simulink model "ee_synrm_torque_control_v1"  (R2023a)
settings: Solver=FixedStepDiscrete  StartTime=0.0  StopTime=1.5  FixedStep=Ts  RelTol=1e-3  EnableMultiTasking=on
PreLoadFcn:
  | ee_synrm_torque_control_data;
StopFcn:
  | ee_addSimlogTimeStamp(bdroot)
undefined symbols (not defined in the file): Ld, Lq, p, Ts
libraries: nesl_utility x13, fl_lib x9, ee_lib x4, eeTransforms x2, eePmsmCurrentController x1, simulink x1, eePwmGeneratorTwoLevel x1, batteryecm_lib x1, SignalEditorBlockLib x1
CloseFcn:
  | clear simlog_ee_synrm_torque_control
  | clear logsout_ee_synrm_torque_control
Description:
  | Synchronous Reluctance Machine Torque Control
settings Model: Creator=The MathWorks, Inc.  LastModifiedBy=ravikrishna_g3
settings SolverCC: AlgebraicLoopSolver=TrustRegion  MaxZcPerStep=1
settings DataIOCC: MaxDataPoints=310000  ReturnWorkspaceOutputs=off  SignalLoggingName=logsout_ee_synrm_torque_control
settings OptimizationCC: ReuseModelBlockBuffer=off  LifeSpan=inf
settings DebuggingCC: UnderspecifiedInitializationDetection=Classic  MergeDetectMultiDrivingBlocksExec=none  UnconnectedInputMsg=warning  UnconnectedOutputMsg=warning  UnconnectedLineMsg=warning  SFUnexpectedBacktrackingDiag=warning  SFNoUnconditionalDefaultTransitionDiag=warning  SFExecutionAtInitializationDiag=none  ArithmeticOperatorsInVariantConditions=warning
settings ModelReferenceCC: EnableRefExpFcnMdlSchedulingChecks=on
settings SFSimCC: SimUseLocalCustomCode=off  CustomCodeUndefinedFunction=UseInterfaceOnly
settings RTWCC: RTWUseLocalCustomCode=off  DLArmComputeVersion=19.05
settings CodeAppCC: StateflowObjectComments=on
settings GRTTargetCC: TargetLangStandard=C89/C90 (ANSI)
settings ConfigComp: CovMetricSettings=dw  CovSaveCumulativeToWorkspaceVar=on  CovSaveSingleToWorkspaceVar=on  CovExternalEMLEnable=off
settings SimscapeCC: SimscapeLogType=all  SimscapeLogSimulationStatistics=on  SimscapeLogName=simlog_ee_synrm_torque_control  SimscapeLogDataHistory=310000

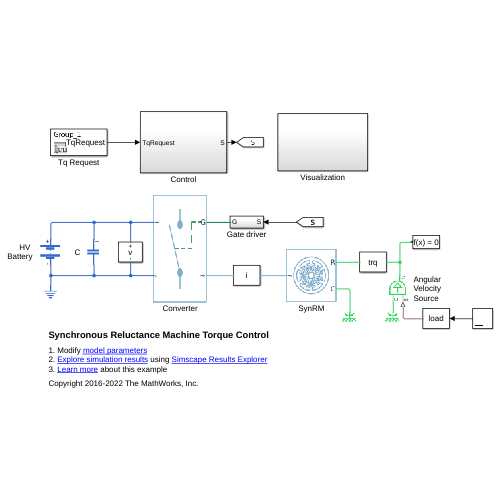
[thumbnail: Simulink's stored preview of the top-level diagram]
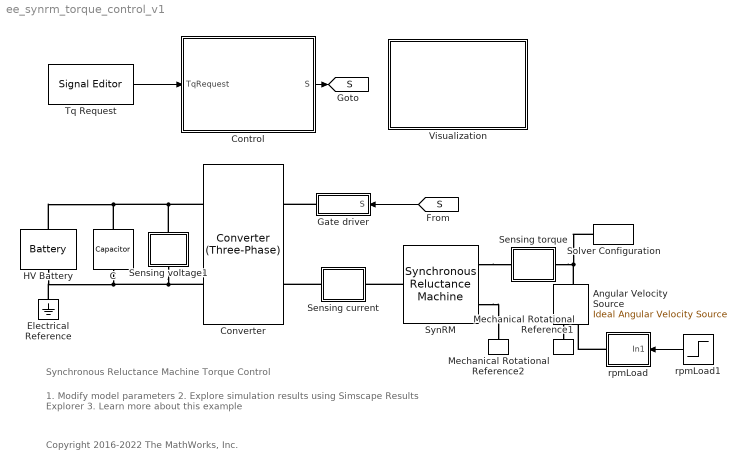
== system ee_synrm_torque_control_v1 ==
  note: Synchronous Reluctance Machine Torque Control
  note: 1. Modify model parameters
      | 2. Explore simulation results using Simscape Results Explorer
      | 3. Learn more about this example
  note: Copyright 2016-2022 The MathWorks, Inc.
  Angular Velocity Source : fl_lib/Mechanical/Mechanical Sources/Ideal Angular Velocity Source
  C : fl_lib/Electrical/Electrical Elements/Capacitor  c=Cdc F  r=1e-6 Ohm  g=0 1/Ohm  i_specify=off  i_priority=None  i=0 A  i_nominal_specify=off  i_nominal_unit=A  i_nominal_value=1  v_specify=off  v_priority=None  v=0 V  v_nominal_specify=off  v_nominal_unit=V  v_nominal_value=1  vc_specify=on  vc_priority=None  vc=Vnom V  vc_nominal_specify=off  vc_nominal_unit=V  vc_nominal_value=1
  Control : Subsystem
  Converter : ee_lib/Semiconductors & Converters/Converters/Converter (Three-Phase)  port_option=ee.enum.threePhasePort.composite  device_type=3  K=0  Vf=0.8 V  Ron=0.001 Ohm  Rds=0.001 Ohm  Goff=1e-5 1/Ohm  Vgt=1 V  Vgt_off=-1 V  Ih=1 A  Vth=0.5 V  diode_param=2  diode_Vf=0.8 V  diode_Ron=0.001 Ohm  diode_Goff=1e-5 1/Ohm  diode_C=50 nF  diode_iRM=-235 A  diode_iF=300 A  diode_idot=-50 A/us  diode_trr_param=1  diode_trr_factor=3  diode_trr=15 us  diode_Qrr=1.5e+3 s*uA  snubber_type=0  Cs=1e-7 F  Rs=0.1 Ohm
  Electrical Reference : fl_lib/Electrical/Electrical Elements/Electrical Reference
  Gate driver : Subsystem
  HV Battery : batteryecm_lib/Battery  Vnom=Vnom V  prm_dir=1  R1_dis=2 Ohm  R1_ch=2 Ohm  R1=0.001 Ohm  prm_AH=1  AH=10000 hr*A  V1=V1 V  AH1=3000 hr*A  prm_R2=1  R2=2000 Ohm  Tmeas=298.15 K  charge_measurement_port=simscape.enum.battery.enable.no  prm_dyn=1  Rp1=0.005 Ohm  tau1=30 s  Rp2=0.005 Ohm  tau2=30 s  Rp3=0.005 Ohm  tau3=30 s  Rp4=0.005 Ohm  tau4=30 s  Rp5=0.005 Ohm  tau5=30 s  prm_fade=1  N_fade=100  AH_fade=45 hr*A  R1_fade=2.02 Ohm  R1_ch_fade=2.02 Ohm  V1_fade=10.35 V  prm_age=1  prm_age_OCV=1  OCV_age=0.9  SOC_age=60  Tmeas_age=298.15 K  delta_time_age_vec=[0] d  temperature_age_vec=[273] K  OCV_scaling_age=2.2134e6  OCV_offset_age=1.632e6  temp_exp_age=0.515833569 V  t_exp_age=0.75  Vnom_T2=12 V  R1_T2=2.2 Ohm  R1_T2_dis=2.2 Ohm  R1_T2_ch=2.2 Ohm  V1_T2=11.4 V  R2_T2=2200 Ohm  Rp1_T2=0.005 Ohm  tau1_T2=30 s  Rp2_T2=0.005 Ohm  tau2_T2=30 s  Rp3_T2=0.005 Ohm  tau3_T2=30 s  Rp4_T2=0.005 Ohm  tau4_T2=30 s  Rp5_T2=0.005 Ohm  tau5_T2=30 s  Tmeas2=273.15 K  thermal_port=simscape.enum.thermaleffects.omit  thermal_mass=30000 J/K  i_specify=off  i_priority=None  i=0 A  i_nominal_specify=off  i_nominal_unit=A  i_nominal_value=1  v_specify=off  v_priority=None  v=0 V  v_nominal_specify=off  v_nominal_unit=V  v_nominal_value=1  charge_specify=on  charge_priority=High  charge=8000 hr*A  charge_nominal_specify=off  charge_nominal_unit=A*hr  charge_nominal_value=1  num_cycles_specify=off  num_cycles_priority=High  num_cycles=0  num_cycles_nominal_specify=off  num_cycles_nominal_unit=1  num_cycles_nominal_value=1  temperature_specify=off  temperature_priority=High  temperature=298.15 K  temperature_nominal_specify=off  temperature_nominal_unit=K  temperature_nominal_value=1
  Mechanical Rotational Reference1 : fl_lib/Mechanical/Rotational Elements/Mechanical Rotational Reference
  Mechanical Rotational Reference2 : fl_lib/Mechanical/Rotational Elements/Mechanical Rotational Reference
  Sensing current : Subsystem
      mask Display: disp('i')
  Sensing torque : Subsystem
      mask Display: disp('trq')
  Sensing voltage1 : Subsystem
      mask Display: disp('v')
  Solver Configuration : nesl_utility/Solver Configuration  PhysicalDomain=network_engine_domain  SubClassName=solver  LeftPortType=input  RightPortType=generic  Tones=[]  Harmonics=[]  SimulateNoise=off  Profile=off  UseLocalSampling=off  EnableSwitchedLinearOptims=on  FrequencyDomain=off  UseCCode=off  RelTol=0.001  AbsTol=1e-06  MinStep=1e-09  ToWorkspace=off  RevertToSquareIcSolve=off  NumHomotopyIterations=100  PhasorMode=off  PhasorModeNumHarmonics=1  ConsistencySolver=NEWTON_FTOL  IndexReductionMethod=DerivativeReplacement  DoDC=off  ResidualTolerance=1e-9  ConsistencyTolSource=GLOBAL  ConsistencyAbsTol=0.001  ConsistencyRelTol=0.001  ConsistencyTolFactor=0.001  UseLocalSolver=on  LocalSolverChoice=NE_BACKWARD_EULER_ADVANCER  ResolveIndetEquations=on  FunctionEvalNumThread=1  LocalSolverSampleTime=Ts  DoFixedCost=on  MaxNonlinIter=5  MaxModeIter=2  ComputeImpulses=off  ImpulseIterations=2  LinearAlgebra=auto  LinearAlgebraNumThread=0  EquationFormulation=NE_TIME_EF  DelaysMemoryBudget=1024  AutomaticFiltering=on  FilteringTimeConstant=0.001  PartitionStorageMethod=AS_NEEDED  PartitionMemoryBudget=1024  PartitionMethod=FAST
  SynRM : ee_lib/Electromechanical/Reluctance & Stepper/Synchronous Reluctance Machine  port_option=ee.enum.threePhasePort.composite  nPolePairs=p  stator_param=1  machine_param=ee.enum.dqparameterization.constant  Ld=Ld H  Lq=Lq H  idVec=[-200, 0, 200] A  iqVec=[-200, 0, 200] A  LdMatrix=0.0031 * ones(3, 3) H  LqMatrix=0.004 * ones(3, 3) H  L0=L0 H  Ls=0.0025 H  Lm=-0.0003 H  Ms=0.0010 H  Rs=Rs Ohm  zero_sequence=ee.enum.park.zerosequence.exclude  iron_loss_option=ee.enum.electromech.synrm.ironloss.specifyRm  Rm=inf Ohm  rotorLossCoeff_k_h_DQ=zeros(3, 3) W/Hz  rotorLossCoeff_k_J_DQ=zeros(3, 3) W/Hz^2  rotorLossCoeff_k_ex_DQ=zeros(3, 3) W/Hz^(3/2)  statorLossCoeff_k_h_DQ=zeros(3, 3) W/Hz  statorLossCoeff_k_J_DQ=zeros(3, 3) W/Hz^2  statorLossCoeff_k_ex_DQ=zeros(3, 3) W/Hz^(3/2)  wVec=[1000, 2000] rpm  rotorLossTable_DQ=zeros(3, 3, 2) W  statorLossTable_DQ=zeros(3, 3, 2) W  J=0 kg*m^2  lam=0 N*m/(rad/s)  axes_param=1  i_d_specify=off  i_d_priority=None  i_d=0 A  i_d_nominal_specify=off  i_d_nominal_unit=A  i_d_nominal_value=1  i_q_specify=off  i_q_priority=None  i_q=0 A  i_q_nominal_specify=off  i_q_nominal_unit=A  i_q_nominal_value=1  torque_specify=off  torque_priority=None  torque=0 N*m  torque_nominal_specify=off  torque_nominal_unit=N*m  torque_nominal_value=1  angular_velocity_specify=off  angular_velocity_priority=High  angular_velocity=0 rpm  angular_velocity_nominal_specify=off  angular_velocity_nominal_unit=rpm  angular_velocity_nominal_value=1  angular_position_specify=off  angular_position_priority=None  angular_position=0 deg  angular_position_nominal_specify=off  angular_position_nominal_unit=deg  angular_position_nominal_value=1  Tmeas=298.15 K  alpha=3.93e-3 1/K  stator_thermal_mass=100 J/K  rotor_thermal_mass=200 J/K  ironloss_percent_rotor=50  temperatureA_specify=off  temperatureA_priority=High  temperatureA=25 degC  temperatureA_nominal_specify=off  temperatureA_nominal_unit=degC  temperatureA_nominal_value=1  temperatureB_specify=off  temperatureB_priority=High  temperatureB=25 degC  temperatureB_nominal_specify=off  temperatureB_nominal_unit=degC  temperatureB_nominal_value=1  temperatureC_specify=off  temperatureC_priority=High  temperatureC=25 degC  temperatureC_nominal_specify=off  temperatureC_nominal_unit=degC  temperatureC_nominal_value=1  temperatureR_specify=off  temperatureR_priority=High  temperatureR=25 degC  temperatureR_nominal_specify=off  temperatureR_nominal_unit=degC  temperatureR_nominal_value=1
      settings: InternalSimscapePortConfiguration="{\"Bottom\":[],\"Left\":[{\"id\":\"N\",\"label\":\"~\",\"type\":\"foundation.electrical.three_phase\"}],\"Right\":[{\"id\":\"R\",\"label\":\"R\",\"type\":\"foundation.mechanical.rotational.rotational\"},{\"id\":\"C\",\"label\":\"C\",\"type\":\"foundation.mechanical.rotational.rotational\"}],\"Top\":[]}"
  Tq Request : SignalEditorBlockLib/Signal Editor  FileName=ee_synrm_torque_control_Tq_Request.mat  ActiveScenario=Group_1  ActiveSignal=TqRequest  IsBus=off  OutputBusObjectStr=Bus: BusObject  SampleTime=0  OutputAfterFinalValue=Extrapolation  Unit=inherit  PreserveSignalName=on  ApplySigPropsToAllScenarios=on
  Visualization : Subsystem
  rpmLoad : Subsystem
      mask Display: disp('load')
  rpmLoad1 : Step  Time=0.05  After=1000  SampleTime=0
  tag scope: S=global
  wires:
  [S] -> Gate driver/1(S)
  rpmLoad1/1 -> rpmLoad/1(In1)
  Control/1(S) -> [S]
  Tq Request/1 -> Control/1(TqRequest)
  connections:
  Angular Velocity Source/LConn1 -- Solver Configuration/RConn1 -- Sensing torque/RConn1
  Angular Velocity Source/RConn2 -- Mechanical Rotational Reference1/LConn1
  Converter/RConn2 -- Sensing voltage1/RConn1 -- Electrical Reference/LConn1 -- HV Battery/RConn1 -- C/RConn1
  Converter/RConn1 -- Sensing voltage1/LConn1 -- HV Battery/LConn1 -- C/LConn1
  Gate driver/RConn1 -- Converter/LConn1
  Sensing current/LConn1 -- Converter/LConn2
  SynRM/LConn1 -- Sensing current/RConn1
  SynRM/RConn1 -- Sensing torque/LConn1
  SynRM/RConn2 -- Mechanical Rotational Reference2/LConn1
  rpmLoad/RConn1 -- Angular Velocity Source/RConn1

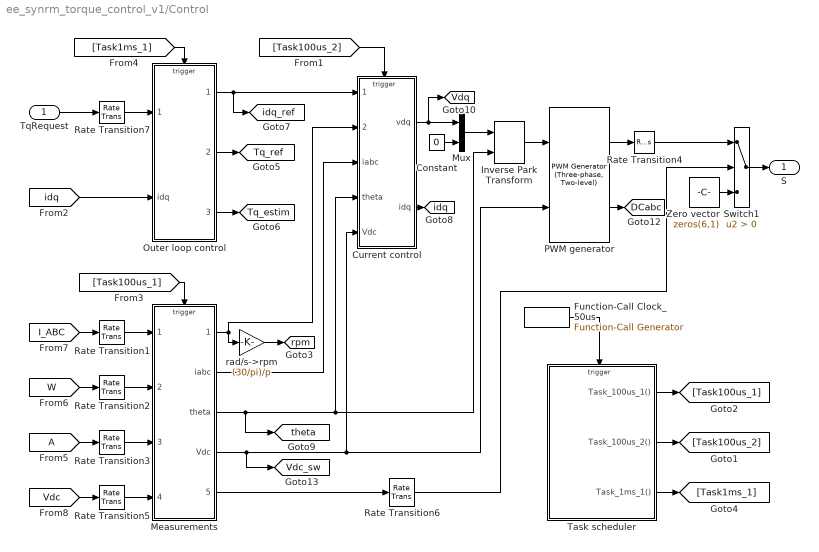
== system ee_synrm_torque_control_v1/Control ==
  TqRequest : Inport
  Constant : Constant  Value=0  SampleTime=-1
  Current control : Subsystem
  From5 : From  TagVisibility=global
  Function-Call Clock_50us : simulink/Ports & Subsystems/Function-Call Generator  sample_time=5e-5  numberOfIterations=1  DisallowWideOutput=off
  Inverse Park Transform : eeTransforms/Inverse Park Transform  AxisAlignment=Q-axis  PowerInvariant=off
  Measurements : Subsystem
  Mux : Mux  Inputs=2
  Outer loop control : Subsystem
  PWM generator : eePwmGeneratorTwoLevel/PWM Generator (Three-phase, Two-level)  PWMMode=Continuous PWM (CPWM)  CPWMMode=SVM: space vector modulation  DPWMMode=60 DPWM: 60 degree discontinuous PWM  fsw=fsw  Ts=Ts
  Rate Transition{1..7} (7 alike) : RateTransition
  Switch1 : Switch  Criteria=u2 > Threshold  SaturateOnIntegerOverflow=off  InputSameDT=off
  Task scheduler : Stateflow chart  TreatAsAtomicUnit=on
  Zero vector : Constant  Value=zeros(6,1)  SampleTime=Ts
  rad/s->rpm : Gain  Gain=(30/pi)/p
  S : Outport  VectorParamsAs1DForOutWhenUnconnected=off
  tag scope: DCabc=global, Tq_estim=global, Tq_ref=global, Vdc_sw=global, Vdq=global, idq=global, idq_ref=global, rpm=global, theta=global
  wires:
  Mux/1 -> Inverse Park Transform/1
  [Vdc] -> Rate Transition5/1
  [W] -> Rate Transition2/1
  TqRequest/1 -> Rate Transition7/1
  Constant/1 -> Mux/2
  Measurements/4(Vdc) -> [Vdc_sw], Current control/5(Vdc), PWM generator/2
  Function-Call Clock_50us/1 -> Task scheduler/Trigger
  Current control/2(idq) -> [idq]
  Switch1/1 -> S/1
  rad/s->rpm/1 -> [rpm]
  Rate Transition7/1 -> Outer loop control/1(TqRequest)
  [Task100us_1] -> Measurements/Trigger
  Inverse Park Transform/1 -> PWM generator/1
  Rate Transition5/1 -> Measurements/4(Vdc_m)
  Zero vector/1 -> Switch1/3
  Measurements/2(iabc) -> Current control/3(iabc)
  Rate Transition6/1 -> Switch1/2
  Rate Transition4/1 -> Switch1/1
  Measurements/5(PwmEnable) -> Rate Transition6/1
  Current control/1(vdq) -> Mux/1, [Vdq]
  PWM generator/1 -> Rate Transition4/1
  Outer loop control/3(Tq_estim) -> [Tq_estim]
  Task scheduler/1(Task_100us_1()) -> [Task100us_1]
  Outer loop control/1(idq_ref) -> [idq_ref], Current control/1(idq_ref)
  [I_ABC] -> Rate Transition1/1
  Measurements/3(theta) -> [theta], Inverse Park Transform/2, Current control/4(theta)
  [idq] -> Outer loop control/2(idq)
  Task scheduler/2(Task_100us_2()) -> [Task100us_2]
  Measurements/1(omega) -> rad/s->rpm/1, Current control/2(omega)
  Outer loop control/2(Tq_ref) -> [Tq_ref]
  Rate Transition2/1 -> Measurements/2(omega_m)
  Task scheduler/3(Task_1ms_1()) -> [Task1ms_1]
  PWM generator/2 -> [DCabc]
  Rate Transition3/1 -> Measurements/3(theta_m)
  Rate Transition1/1 -> Measurements/1(iabc_m)
  From5/1 -> Rate Transition3/1
  [Task1ms_1] -> Outer loop control/Trigger
  [Task100us_2] -> Current control/Trigger

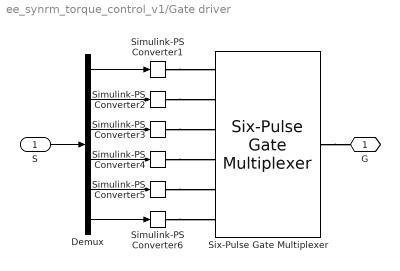
== system ee_synrm_torque_control_v1/Gate driver ==
  S : Inport
  Demux : Demux  Outputs=6
  Simulink-PS Converter{1..6} (6 alike) : nesl_utility/Simulink-PS Converter  PhysicalDomain=network_engine_domain  SubClassName=ps_input  LeftPortType=input  RightPortType=output  PseudoPeriodic=off  Frequencies=[]  NoiseDistribution=none  NoiseParameters=[]  Unit=1  AffineConversion=off  FilteringAndDerivatives=zero  SimscapeFilterOrder=1  InputFilterTimeConstant=0.001  UdotUserProvided=1
  Six-Pulse Gate Multiplexer : ee_lib/Semiconductors & Converters/Converters/Six-Pulse Gate Multiplexer  port_option=ee.enum.controlport.ps
  G : PMIOPort  Side=Right
  wires:
  Demux/1 -> Simulink-PS Converter1/1
  S/1 -> Demux/1
  Demux/4 -> Simulink-PS Converter4/1
  Demux/2 -> Simulink-PS Converter2/1
  Demux/3 -> Simulink-PS Converter3/1
  Demux/5 -> Simulink-PS Converter5/1
  Demux/6 -> Simulink-PS Converter6/1
  connections:
  Six-Pulse Gate Multiplexer/RConn1 -- G/RConn1
  Simulink-PS Converter1/RConn1 -- Six-Pulse Gate Multiplexer/LConn1
  Simulink-PS Converter3/RConn1 -- Six-Pulse Gate Multiplexer/LConn3
  Simulink-PS Converter5/RConn1 -- Six-Pulse Gate Multiplexer/LConn5
  Simulink-PS Converter6/RConn1 -- Six-Pulse Gate Multiplexer/LConn6
  Simulink-PS Converter4/RConn1 -- Six-Pulse Gate Multiplexer/LConn4
  Simulink-PS Converter2/RConn1 -- Six-Pulse Gate Multiplexer/LConn2

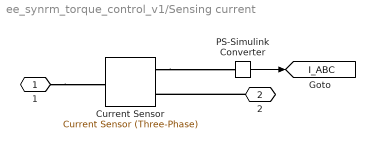
== system ee_synrm_torque_control_v1/Sensing current ==
  Current Sensor : ee_lib/Sensors & Transducers/Current Sensor (Three-Phase)
  PS-Simulink Converter : nesl_utility/PS-Simulink Converter  PhysicalDomain=network_engine_domain  SubClassName=ps_output  LeftPortType=input  RightPortType=output  PseudoPeriodic=off  Frequencies=[]  VectorFormat=1-D array  Unit=A  AffineConversion=off
  1 : PMIOPort  Side=Left
  2 : PMIOPort  Port=2  Side=Right
  tag scope: I_ABC=global
  wires:
  PS-Simulink Converter/1 -> [I_ABC]
  connections:
  1/RConn1 -- Current Sensor/LConn1
  2/RConn1 -- Current Sensor/RConn2
  Current Sensor/RConn1 -- PS-Simulink Converter/LConn1

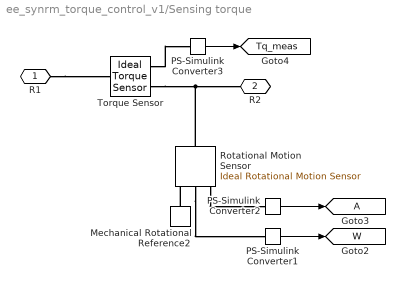
== system ee_synrm_torque_control_v1/Sensing torque ==
  Goto3 : Goto  TagVisibility=global
  Mechanical Rotational Reference2 : fl_lib/Mechanical/Rotational Elements/Mechanical Rotational Reference
  PS-Simulink Converter1 : nesl_utility/PS-Simulink Converter  PhysicalDomain=network_engine_domain  SubClassName=ps_output  LeftPortType=input  RightPortType=output  PseudoPeriodic=off  Frequencies=[]  VectorFormat=1-D array  Unit=rad/s  AffineConversion=off
  PS-Simulink Converter2 : nesl_utility/PS-Simulink Converter  PhysicalDomain=network_engine_domain  SubClassName=ps_output  LeftPortType=input  RightPortType=output  PseudoPeriodic=off  Frequencies=[]  VectorFormat=1-D array  Unit=rad  AffineConversion=off
  PS-Simulink Converter3 : nesl_utility/PS-Simulink Converter  PhysicalDomain=network_engine_domain  SubClassName=ps_output  LeftPortType=input  RightPortType=output  PseudoPeriodic=off  Frequencies=[]  VectorFormat=1-D array  Unit=N*m  AffineConversion=off
  Rotational Motion Sensor : fl_lib/Mechanical/Mechanical Sensors/Ideal Rotational Motion Sensor  reference=foundation.enum.MeasurementReference.difference  acceleration_port=false  velocity_port=true  position_port=true  wrap_angle=simscape.enum.onoff.off  offset=0 deg
  Torque Sensor : fl_lib/Mechanical/Mechanical Sensors/Ideal Torque Sensor
  R1 : PMIOPort  Side=Left
  R2 : PMIOPort  Port=2  Side=Right
  tag scope: Tq_meas=global, W=global
  wires:
  PS-Simulink Converter3/1 -> [Tq_meas]
  PS-Simulink Converter1/1 -> [W]
  PS-Simulink Converter2/1 -> Goto3/1
  connections:
  R1/RConn1 -- Torque Sensor/LConn1
  Torque Sensor/RConn2 -- PS-Simulink Converter3/LConn1
  Torque Sensor/RConn1 -- Rotational Motion Sensor/LConn1 -- R2/RConn1
  Rotational Motion Sensor/RConn3 -- PS-Simulink Converter2/LConn1
  Rotational Motion Sensor/RConn2 -- PS-Simulink Converter1/LConn1
  Mechanical Rotational Reference2/LConn1 -- Rotational Motion Sensor/RConn1

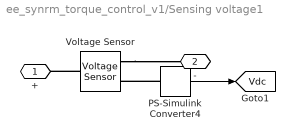
== system ee_synrm_torque_control_v1/Sensing voltage1 ==
  PS-Simulink Converter4 : nesl_utility/PS-Simulink Converter  PhysicalDomain=network_engine_domain  SubClassName=ps_output  LeftPortType=input  RightPortType=output  PseudoPeriodic=off  Frequencies=[]  VectorFormat=1-D array  Unit=V  AffineConversion=off
  Voltage Sensor : fl_lib/Electrical/Electrical Sensors/Voltage Sensor
  + : PMIOPort  Side=Left
  - : PMIOPort  Port=2  Side=Right
  tag scope: Vdc=global
  wires:
  PS-Simulink Converter4/1 -> [Vdc]
  connections:
  Voltage Sensor/LConn1 -- +/RConn1
  Voltage Sensor/RConn2 -- -/RConn1
  PS-Simulink Converter4/LConn1 -- Voltage Sensor/RConn1

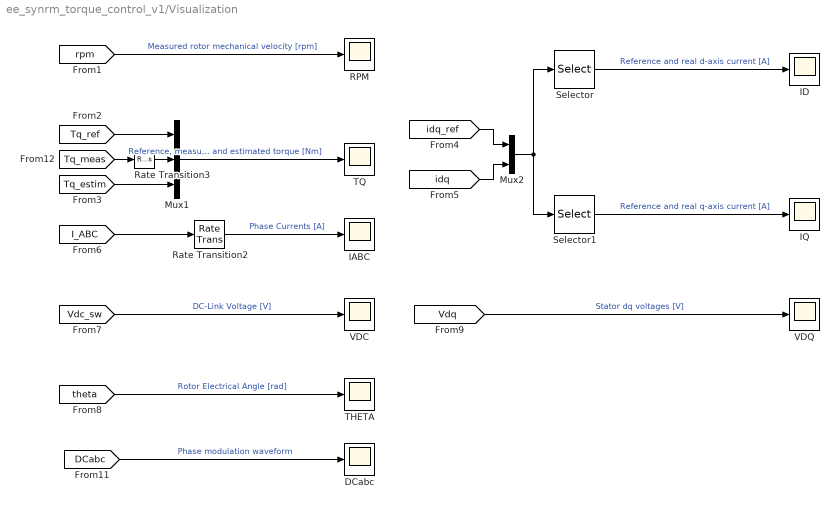
== system ee_synrm_torque_control_v1/Visualization ==
  DCabc : Scope
  IABC : Scope
  ID : Scope
  IQ : Scope
  Mux1 : Mux  Inputs=3
  Mux2 : Mux  Inputs=2
  RPM : Scope
  Rate Transition2 : RateTransition  OutPortSampleTime=1e-4
  Rate Transition3 : RateTransition
  Selector : Selector  InputPortWidth=4  IndexOptions=Index vector (dialog)  Indices=[1 3]  OutputSizes=1
  Selector1 : Selector  InputPortWidth=4  IndexOptions=Index vector (dialog)  Indices=[2 4]  OutputSizes=1
  THETA : Scope
  TQ : Scope
  VDC : Scope
  VDQ : Scope
  wires:
  Rate Transition3/1 -> Mux1/2
  [Tq_meas] -> Rate Transition3/1
  [Vdc_sw] -> VDC/1  "DC-Link Voltage [V]"
  [I_ABC] -> Rate Transition2/1
  [Tq_estim] -> Mux1/3
  [theta] -> THETA/1  "Rotor Electrical Angle [rad]"
  Selector/1 -> ID/1  "Reference and real d-axis current [A]"
  [Vdq] -> VDQ/1  "Stator dq voltages [V]"
  Mux2/1 -> Selector1/1, Selector/1
  Selector1/1 -> IQ/1  "Reference and real q-axis current [A]"
  [idq_ref] -> Mux2/1
  Mux1/1 -> TQ/1  "Reference, measured and estimated torque [Nm]"
  [DCabc] -> DCabc/1  "Phase modulation waveform"
  [rpm] -> RPM/1  "Measured rotor mechanical velocity [rpm]"
  [Tq_ref] -> Mux1/1
  Rate Transition2/1 -> IABC/1  "Phase Currents [A]"
  [idq] -> Mux2/2

== system ee_synrm_torque_control_v1/rpmLoad ==
  In1 : Inport
  Rate limiter 10000rpm/s : RateLimiter  RisingSlewLimit=10000  FallingSlewLimit=-10000  SampleTimeMode=inherited
  Simulink-PS Converter : nesl_utility/Simulink-PS Converter  PhysicalDomain=network_engine_domain  SubClassName=ps_input  LeftPortType=input  RightPortType=output  PseudoPeriodic=off  Frequencies=[]  NoiseDistribution=none  NoiseParameters=[]  Unit=rpm  AffineConversion=off  FilteringAndDerivatives=zero  SimscapeFilterOrder=1  InputFilterTimeConstant=0.001  UdotUserProvided=1
  Conn1 : PMIOPort  Side=Right
  wires:
  Rate limiter 10000rpm/s/1 -> Simulink-PS Converter/1
  In1/1 -> Rate limiter 10000rpm/s/1
  connections:
  Simulink-PS Converter/RConn1 -- Conn1/RConn1

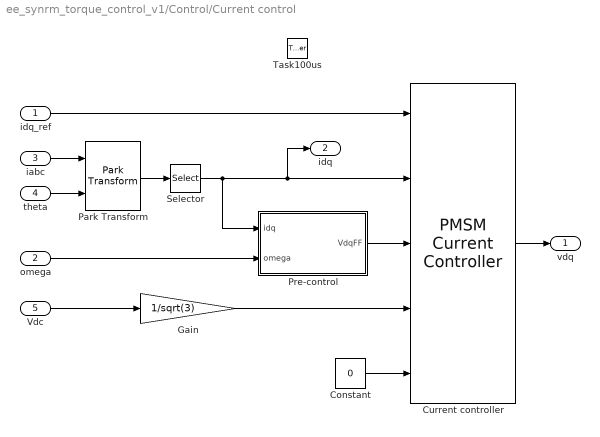
== system ee_synrm_torque_control_v1/Control/Current control ==
  idq_ref : Inport
  omega : Inport  Port=2
  iabc : Inport  Port=3
  theta : Inport  Port=4
  Vdc : Inport  Port=5
  Task100us : TriggerPort  TriggerType=function-call  VariantControl=Variant  PortDimensions=1
  Constant : Constant  Value=0  SampleTime=-1
  Current controller : eePmsmCurrentController/PMSM Current Controller  Kp_id=Kp_id  Ki_id=Ki_id  Kaw_id=1  Kp_iq=Kp_iq  Ki_iq=Ki_iq  Kaw_iq=1  Ts=-1  Tsd=Tsi  AxisPrio=Q-axis  ActZC=on  ActFF=on
  Gain : Gain  Gain=1/sqrt(3)
  Park Transform : eeTransforms/Park Transform  AxisAlignment=Q-axis  PowerInvariant=off
  Pre-control : Subsystem
  Selector : Selector  InputPortWidth=3  IndexOptions=Index vector (dialog)  Indices=[1 2]  OutputSizes=1
  vdq : Outport  VectorParamsAs1DForOutWhenUnconnected=off
  idq : Outport  Port=2  VectorParamsAs1DForOutWhenUnconnected=off
  wires:
  theta/1 -> Park Transform/2
  Gain/1 -> Current controller/4
  iabc/1 -> Park Transform/1
  idq_ref/1 -> Current controller/1
  Vdc/1 -> Gain/1
  Constant/1 -> Current controller/5
  Park Transform/1 -> Selector/1
  Current controller/1 -> vdq/1
  Pre-control/1(VdqFF) -> Current controller/3
  Selector/1 -> Pre-control/1(idq), idq/1, Current controller/2
  omega/1 -> Pre-control/2(omega)

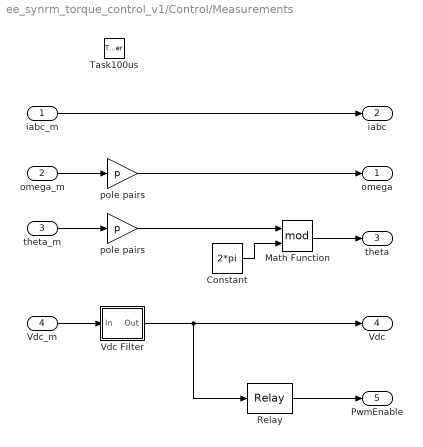
== system ee_synrm_torque_control_v1/Control/Measurements ==
  iabc_m : Inport
  omega_m : Inport  Port=2
  theta_m : Inport  Port=3
  Vdc_m : Inport  Port=4
  Task100us : TriggerPort  TriggerType=function-call  VariantControl=Variant  PortDimensions=1
  Constant : Constant  Value=2*pi  SampleTime=-1
  Math Function : Math  Operator=mod  SignedPower=on
  Relay : Relay  OnSwitchValue=100  OffSwitchValue=50
  Vdc Filter : Subsystem  mask(Discrete first-order filter (Low-pass)){T=0.005, Ts=1e-4}
      mask prompts: T "Time constant (s):"; Ts "Sample time (s):"
      mask help: This block implements a discrete low-pass filter. To calculate the coefficients, the block discretises a continuous low-pass filter using the Tustin method.
      mask init:
      | num = [ Ts/(2*T + Ts), Ts/(2*T + Ts)];
      | den = [ 1, -(2*T - Ts)/(2*T + Ts)];
  pole pairs : Gain  Gain=p
  "pole pairs " : Gain  Gain=p
  omega : Outport  VectorParamsAs1DForOutWhenUnconnected=off
  iabc : Outport  Port=2  VectorParamsAs1DForOutWhenUnconnected=off
  theta : Outport  Port=3  VectorParamsAs1DForOutWhenUnconnected=off
  Vdc : Outport  Port=4  VectorParamsAs1DForOutWhenUnconnected=off
  PwmEnable : Outport  Port=5  VectorParamsAs1DForOutWhenUnconnected=off
  wires:
  pole pairs/1 -> omega/1
  Vdc_m/1 -> Vdc Filter/1(In)
  theta_m/1 -> "pole pairs "/1
  omega_m/1 -> pole pairs/1
  iabc_m/1 -> iabc/1
  "pole pairs "/1 -> Math Function/1
  Constant/1 -> Math Function/2
  Math Function/1 -> theta/1
  Relay/1 -> PwmEnable/1
  Vdc Filter/1(Out) -> Relay/1, Vdc/1

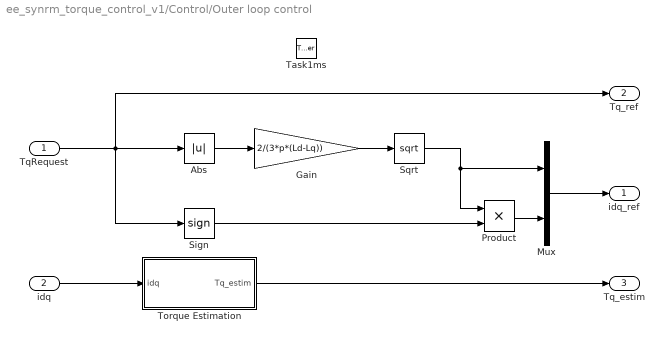
== system ee_synrm_torque_control_v1/Control/Outer loop control ==
  TqRequest : Inport
  idq : Inport  Port=2
  Task1ms : TriggerPort  TriggerType=function-call  VariantControl=Variant  PortDimensions=1
  Abs : Abs  SaturateOnIntegerOverflow=off
  Gain : Gain  Gain=2/(3*p*(Ld-Lq))
  Mux : Mux  Inputs=2
  Product : Product
  Sign : Signum
  Sqrt : Sqrt
  Torque Estimation : Subsystem
  idq_ref : Outport  VectorParamsAs1DForOutWhenUnconnected=off
  Tq_ref : Outport  Port=2  VectorParamsAs1DForOutWhenUnconnected=off
  Tq_estim : Outport  Port=3  VectorParamsAs1DForOutWhenUnconnected=off
  wires:
  Mux/1 -> idq_ref/1
  idq/1 -> Torque Estimation/1(idq)
  TqRequest/1 -> Tq_ref/1, Sign/1, Abs/1
  Abs/1 -> Gain/1
  Gain/1 -> Sqrt/1
  Sqrt/1 -> Product/1, Mux/1
  Product/1 -> Mux/2
  Torque Estimation/1(Tq_estim) -> Tq_estim/1
  Sign/1 -> Product/2

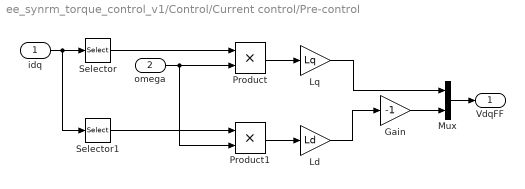
== system ee_synrm_torque_control_v1/Control/Current control/Pre-control ==
  idq : Inport
  omega : Inport  Port=2
  Gain : Gain  Gain=-1
  Ld : Gain  Gain=Ld
  Lq : Gain  Gain=Lq
  Mux : Mux  Inputs=2
  Product : Product
  Product1 : Product
  Selector : Selector  InputPortWidth=2  IndexOptions=Index vector (dialog)  Indices=2  OutputSizes=1
  Selector1 : Selector  InputPortWidth=2  IndexOptions=Index vector (dialog)  Indices=1  OutputSizes=1
  VdqFF : Outport  VectorParamsAs1DForOutWhenUnconnected=off
  wires:
  Product1/1 -> Ld/1
  omega/1 -> Product1/2, Product/2
  Product/1 -> Lq/1
  idq/1 -> Selector1/1, Selector/1
  Lq/1 -> Mux/1
  Ld/1 -> Gain/1
  Mux/1 -> VdqFF/1
  Gain/1 -> Mux/2
  Selector/1 -> Product/1
  Selector1/1 -> Product1/1

== system ee_synrm_torque_control_v1/Control/Measurements/Vdc Filter ==
  In : Inport
  Discrete Transfer Fcn : DiscreteTransferFcn  Numerator=num  Denominator=den
  Out : Outport  VectorParamsAs1DForOutWhenUnconnected=off
  wires:
  Discrete Transfer Fcn/1 -> Out/1
  In/1 -> Discrete Transfer Fcn/1

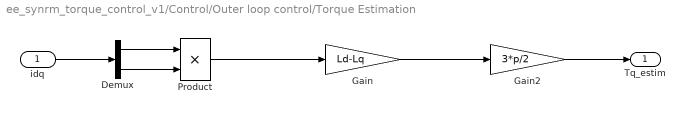
== system ee_synrm_torque_control_v1/Control/Outer loop control/Torque Estimation ==
  idq : Inport
  Demux : Demux  Outputs=2
  Gain : Gain  Gain=Ld-Lq
  Gain2 : Gain  Gain=3*p/2
  Product : Product
  Tq_estim : Outport  VectorParamsAs1DForOutWhenUnconnected=off
  wires:
  idq/1 -> Demux/1
  Demux/1 -> Product/1
  Product/1 -> Gain/1
  Demux/2 -> Product/2
  Gain/1 -> Gain2/1
  Gain2/1 -> Tq_estim/1

== stateflow chart ee_synrm_torque_control_v1/Control/Task scheduler ==
  (default) -> (junction 23) : CLK_50us
  (junction 23) -> (junction 17)
  (junction 17) -> (junction 22) [order 2]
  (junction 17) -> (junction 22) [order 1] : [cnt%%2==0]{Task_100us_1;}
  (junction 22) -> (junction 18) [order 2]
  (junction 22) -> (junction 18) [order 1] : [cnt%%2==0]{Task_100us_2;}
  (junction 18) -> (junction 21) [order 1] : [cnt%%20==0]{Task_1ms_1;}
  (junction 18) -> (junction 21) [order 2]
  (junction 21) -> (junction 34) [order 2]
  (junction 21) -> (junction 16) [order 1] : [1]{cnt++;}
  data: cnt local int32
  events: Task_100us_1 output FUNCTION_CALL_EVENT; Task_100us_2 output FUNCTION_CALL_EVENT; Task_1ms_1 output FUNCTION_CALL_EVENT; CLK_50us input FUNCTION_CALL_EVENT
